simulink model "MEKFTester"  (R2025b)
settings: Solver=VariableStepAuto  StartTime=0.0  StopTime=2000  RelTol=1e-3
values from neighbouring files (symbols this model uses):
  F = StateTransitionMat(z(1:3), z(4:6), R_b2i)    [EstimateStateFCN.m]    (also in FlightEstimator.m = StateTransitionMat(z(1:3), z(4:6), R_b2i, 0); GroundEstimator.m = StateTransitionMat(z(1:3), z(4:6), R_b2i, 1); StateTransitionMat.m = zeros(15))
  q = q / norm(q)    [EstimateStateFCN.m]    (also in FlightEstimator.m; GroundEstimator.m)
undefined symbols (not defined in the file or in its folder): constantsASTRA, DiscIntNeverNeededParam, distMode, dt_SIM, IMU_Rate, Light, magDistMatrix, MIL, u0, x0
libraries: aerolibnav x2, aerolibwind2 x1, simulink x1
settings Model: PacingRate=5  Creator=antho  LastModifiedBy=pplat

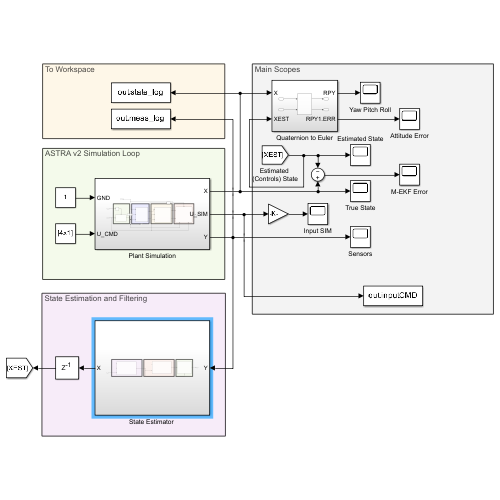
[thumbnail: Simulink's stored preview of the top-level diagram]
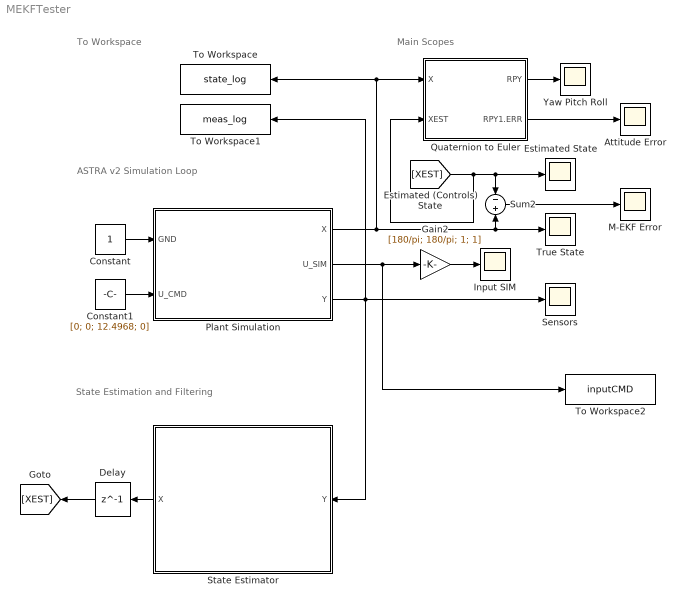
== system MEKFTester ==
  note: To Workspace
  note: Main Scopes
  note: State Estimation and Filtering
  note: ASTRA v2 Simulation Loop
  Attitude Error : Scope
      settings: ActiveDisplayYMinimum=-3.1070378293328353  ActiveDisplayYMaximum=3.3991083276723568  DataLoggingVariableName=ScopeData9
  Constant : Constant
  Constant1 : Constant  Value=[0; 0; 12.4968; 0]
  Delay : Delay  DelayLength=1  InitialCondition=[1; zeros(18,1)]
  Estimated State : Scope
      settings: ActiveDisplayYMinimum=0.77321879382653858  ActiveDisplayYMaximum=0.79869453057358752
  Gain2 : Gain  Gain=[180/pi; 180/pi; 1; 1]
  Input SIM : Scope
      settings: ActiveDisplayYMinimum=-0.41301379982025921  ActiveDisplayYMaximum=0.5556666783325932  DataLoggingVariableName=ScopeData4
  M-EKF Error : Scope
      settings: ActiveDisplayYMinimum=-0.21315959179084651  ActiveDisplayYMaximum=0.079913819904229133  DataLoggingVariableName=ScopeData2
  Plant Simulation : Subsystem
  Quaternion to Euler : Subsystem
  Sensors : Scope
      settings: ActiveDisplayYMinimum=-2.5727575775910978  ActiveDisplayYMaximum=2.4937672733000804  DataLoggingVariableName=ScopeData3
  "State Estimator " : Subsystem
  Sum2 : Sum  Inputs=-|+
  To Workspace : ToWorkspace  VariableName=state_log  SaveFormat=Timeseries  SampleTime=-1
  To Workspace1 : ToWorkspace  VariableName=meas_log  SaveFormat=Timeseries  SampleTime=-1
  To Workspace2 : ToWorkspace  VariableName=inputCMD  SaveFormat=Timeseries  SampleTime=-1
  True State : Scope
      settings: ActiveDisplayYMinimum=-1.2379536808786333  ActiveDisplayYMaximum=1.2486615200976259
  Yaw Pitch Roll : Scope
      settings: ActiveDisplayYMinimum=-224.99023889502547  ActiveDisplayYMaximum=224.99733749831469  DataLoggingVariableName=ScopeData7
  wires:
  [XEST] -> Quaternion to Euler/2(XEST), Sum2/1, Estimated State/1
  Sum2/1 -> M-EKF Error/1
  Delay/1 -> [XEST]
  Gain2/1 -> Input SIM/1
  Plant Simulation/2(U_SIM) -> To Workspace2/1, Gain2/1
  Quaternion to Euler/1(RPY) -> Yaw Pitch Roll/1
  Plant Simulation/3(Y) -> Sensors/1, "State Estimator "/1(Y), To Workspace1/1
  Plant Simulation/1(X) -> Sum2/2, True State/1, Quaternion to Euler/1(X), To Workspace/1
  Constant/1 -> Plant Simulation/1(GND)
  Constant1/1 -> Plant Simulation/2(U_CMD)
  "State Estimator "/1(X) -> Delay/1
  Quaternion to Euler/2(RPY1.ERR) -> Attitude Error/1

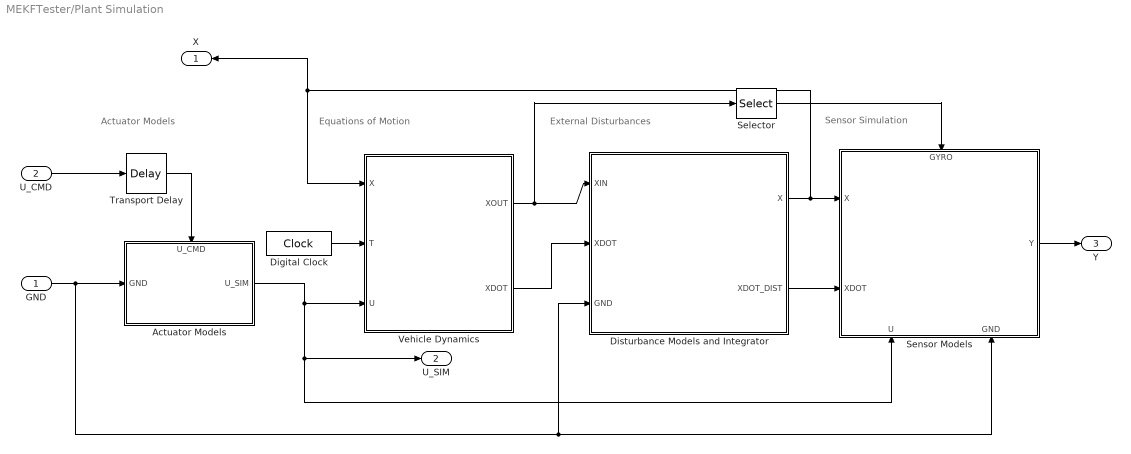
== system MEKFTester/Plant Simulation ==
  note: Equations of Motion
  note: Actuator Models
  note: External Disturbances
  note: Sensor Simulation
  GND : Inport
  U_CMD : Inport  Port=2
  Actuator Models : Subsystem
      settings: PortSchema="{\"entries\":[{\"content\":{\"sides\":[{\"content\":{\"connectorIds\":[\"In1\"]},\"type\":\"ConnectorPlacement.EquallySpacedRectSide\",\"uuid\":\"54343072-6023-41e9-a0f6-81f6bed17e05\"},{\"content\":{\"connectorIds\":[\"Out1\"],\"side\":\"RIGHT\"},\"type\":\"ConnectorPlacement.EquallySpacedRectSide\",\"uuid\":\"2ed3290f-d38b-41d8-95ae-d88068502334\"},{\"content\":{\"connectorIds\":[\"In2\"],\"side\":\"TOP\"},\"type\":\"ConnectorPlacement.EquallySpacedRectSide\",\"uuid\":\"e9e41c57-b871-4be2-92e8-dfbbf995d6b0\"}]},\"type\":\"ConnectorPlacement.EquallySpacedConnector\",\"uuid\":\"c037521e-b20b-40c6-bb74-3aafe8fc1476\"}],\"packageUris\":[\"http://schema.mathworks.com/mf0/Connector/R2020b\"],\"version\":\"1.0\"}"
  Digital Clock : DigitalClock  SampleTime=dt_SIM
  Disturbance Models and Integrator : Subsystem
  Selector : Selector  InputPortWidth=19  IndexOptions=Index vector (dialog)  Indices=[11:13]  OutputSizes=1
  Sensor Models : Subsystem
      settings: PortSchema="{\"entries\":[{\"content\":{\"sides\":[{\"content\":{\"connectorIds\":[\"In1\",\"In2\"]},\"type\":\"ConnectorPlacement.EquallySpacedRectSide\",\"uuid\":\"9bc4a206-bba4-4c50-88a9-89b0392ab722\"},{\"content\":{\"connectorIds\":[\"Out1\"],\"side\":\"RIGHT\"},\"type\":\"ConnectorPlacement.EquallySpacedRectSide\",\"uuid\":\"162bbd17-e1b8-4f29-9191-53e17e38d79d\"},{\"content\":{\"connectorIds\":[\"In3\"],\"side\":\"TOP\"},\"type\":\"ConnectorPlacement.EquallySpacedRectSide\",\"uuid\":\"c56a23db-6a5c-435f-99fd-d50fc9dbdc94\"},{\"content\":{\"connectorIds\":[\"In4\",\"In5\"],\"side\":\"BOTTOM\"},\"type\":\"ConnectorPlacement.EquallySpacedRectSide\",\"uuid\":\"e0c2a0dc-3b7a-40ac-8345-28e7bf7b9405\"}]},\"type\":\"ConnectorPlacement.EquallySpacedConnector\",\"uuid\":\"d1c29f55-9be5-4f45-9d70-06beba2c2f44\"}],\"packageUris\":[\"http://schema.mathworks.com/mf0/Connector/R2020b\"],\"version\":\"1.0\"}"
  Transport Delay : TransportDelay  DelayTime=0.02  InitialOutput=u0
  Vehicle Dynamics : Subsystem
  X : Outport
  U_SIM : Outport  Port=2
  Y : Outport  Port=3
  wires:
  Vehicle Dynamics/2(XDOT) -> Disturbance Models and Integrator/2(XDOT)
  Sensor Models/1(Y) -> Y/1
  GND/1 -> Actuator Models/1(GND), Sensor Models/5(GND), Disturbance Models and Integrator/3(GND)
  Disturbance Models and Integrator/1(X) -> Vehicle Dynamics/1(X), X/1, Sensor Models/1(X)
  Disturbance Models and Integrator/2(XDOT_DIST) -> Sensor Models/2(XDOT)
  Actuator Models/1(U_SIM) -> U_SIM/1, Sensor Models/4(U), Vehicle Dynamics/3(U)
  U_CMD/1 -> Transport Delay/1
  Transport Delay/1 -> Actuator Models/2(U_CMD)
  Vehicle Dynamics/1(XOUT) -> Selector/1, Disturbance Models and Integrator/1(XIN)
  Digital Clock/1 -> Vehicle Dynamics/2(T)
  Selector/1 -> Sensor Models/3(GYRO)

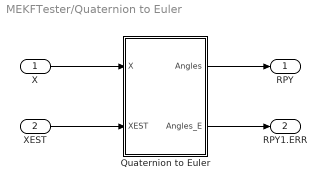
== system MEKFTester/Quaternion to Euler ==
  X : Inport
  XEST : Inport  Port=2
  Quaternion to Euler : MATLAB Function  TreatAsAtomicUnit=on
  RPY : Outport
  RPY1.ERR : Outport  Port=2
  wires:
  X/1 -> Quaternion to Euler/1(X)
  Quaternion to Euler/1(Angles) -> RPY/1
  XEST/1 -> Quaternion to Euler/2(XEST)
  Quaternion to Euler/2(Angles_E) -> RPY1.ERR/1

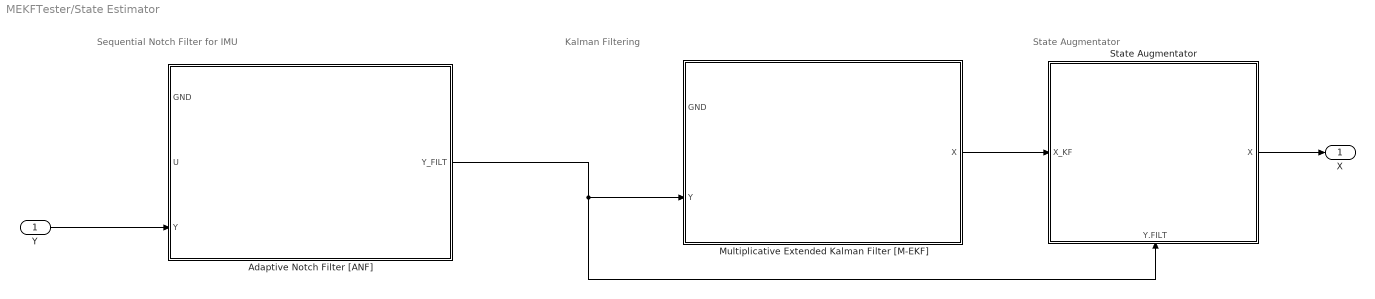
== system MEKFTester/State Estimator  ==
  note: Sequential Notch Filter for IMU
  note: State Augmentator
  note: Kalman Filtering
  Y : Inport
  Adaptive Notch Filter [ANF] : Subsystem
  Multiplicative Extended Kalman Filter [M-EKF] : Subsystem
  State Augmentator : Subsystem
      settings: PortSchema="{\"entries\":[{\"content\":{\"sides\":[{\"content\":{\"connectorIds\":[\"In1\"]},\"type\":\"ConnectorPlacement.EquallySpacedRectSide\",\"uuid\":\"bb6458aa-622a-4d42-b468-f616d6e302fe\"},{\"content\":{\"connectorIds\":[\"Out1\"],\"side\":\"RIGHT\"},\"type\":\"ConnectorPlacement.EquallySpacedRectSide\",\"uuid\":\"af8bade2-eb0a-4714-9db5-d33244eb3558\"},{\"content\":{\"side\":\"TOP\"},\"type\":\"ConnectorPlacement.EquallySpacedRectSide\",\"uuid\":\"05a7f106-e447-475e-b3b5-727cb0579a7b\"},{\"content\":{\"connectorIds\":[\"In2\"],\"side\":\"BOTTOM\"},\"type\":\"ConnectorPlacement.EquallySpacedRectSide\",\"uuid\":\"a6d44455-a42d-44f7-b37b-0d3db398c8f2\"}]},\"type\":\"ConnectorPlacement.EquallySpacedConnector\",\"uuid\":\"c6f62579-6b17-43b5-92f1-6190f0d9fd8b\"}],\"packageUris\":[\"http://schema.mathworks.com/mf0/Connector/R2020b\"],\"version\":\"1.0\"}"
  X : Outport
  wires:
  Multiplicative Extended Kalman Filter [M-EKF]/1(X) -> State Augmentator/1(X_KF)
  State Augmentator/1(X) -> X/1
  Adaptive Notch Filter [ANF]/1(Y_FILT) -> State Augmentator/2(Y.FILT), Multiplicative Extended Kalman Filter [M-EKF]/2(Y)
  Y/1 -> Adaptive Notch Filter [ANF]/3(Y)

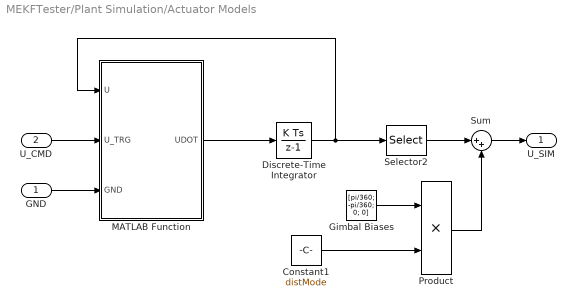
== system MEKFTester/Plant Simulation/Actuator Models ==
  GND : Inport
  U_CMD : Inport  Port=2
  Constant1 : Constant  Value=distMode
  Discrete-Time Integrator : DiscreteIntegrator  InitialCondition=[zeros(4,1); u0(3); 0]  SampleTime=-1  ICPrevOutput=DiscIntNeverNeededParam  ICPrevScaledInput=DiscIntNeverNeededParam
  Gimbal Biases : Constant  Value=[pi/360; -pi/360; 0; 0]
  MATLAB Function : MATLAB Function  TreatAsAtomicUnit=on
  Product : Product
  Selector2 : Selector  InputPortWidth=6  IndexOptions=Index vector (dialog)  Indices=[1 3 5 6]  OutputSizes=1
  Sum : Sum  Inputs=|++
  U_SIM : Outport
  wires:
  U_CMD/1 -> MATLAB Function/2(U_TRG)
  MATLAB Function/1(UDOT) -> Discrete-Time Integrator/1
  Discrete-Time Integrator/1 -> MATLAB Function/1(U), Selector2/1
  GND/1 -> MATLAB Function/3(GND)
  Sum/1 -> U_SIM/1
  Selector2/1 -> Sum/1
  Gimbal Biases/1 -> Product/1
  Product/1 -> Sum/2
  Constant1/1 -> Product/2

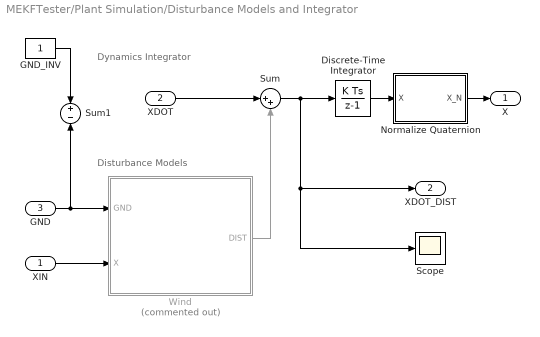
== system MEKFTester/Plant Simulation/Disturbance Models and Integrator ==
  note: Disturbance Models
  note: Dynamics Integrator
  XIN : Inport
  XDOT : Inport  Port=2
  GND : Inport  Port=3
  Discrete-Time Integrator : DiscreteIntegrator  InitialCondition=[x0; zeros(3,1)]  SampleTime=-1  ICPrevOutput=DiscIntNeverNeededParam  ICPrevScaledInput=DiscIntNeverNeededParam
  GND_INV : Constant
  Normalize Quaternion : MATLAB Function  TreatAsAtomicUnit=on
  Scope : Scope
      settings: ActiveDisplayYMinimum=-1  ActiveDisplayYMaximum=1  DataLoggingVariableName=ScopeData8
  Sum : Sum  Inputs=|++
  Sum1 : Sum  Inputs=+|-
  Wind : Subsystem  Commented=on
  X : Outport
  XDOT_DIST : Outport  Port=2
  wires:
  Discrete-Time Integrator/1 -> Normalize Quaternion/1(X)
  XIN/1 -> Wind/2(X)
  Wind/1(DIST) -> Sum/2
  GND_INV/1 -> Sum1/1
  GND/1 -> Wind/1(GND), Sum1/2
  XDOT/1 -> Sum/1
  Sum/1 -> Discrete-Time Integrator/1, Scope/1, XDOT_DIST/1
  Normalize Quaternion/1(X_N) -> X/1

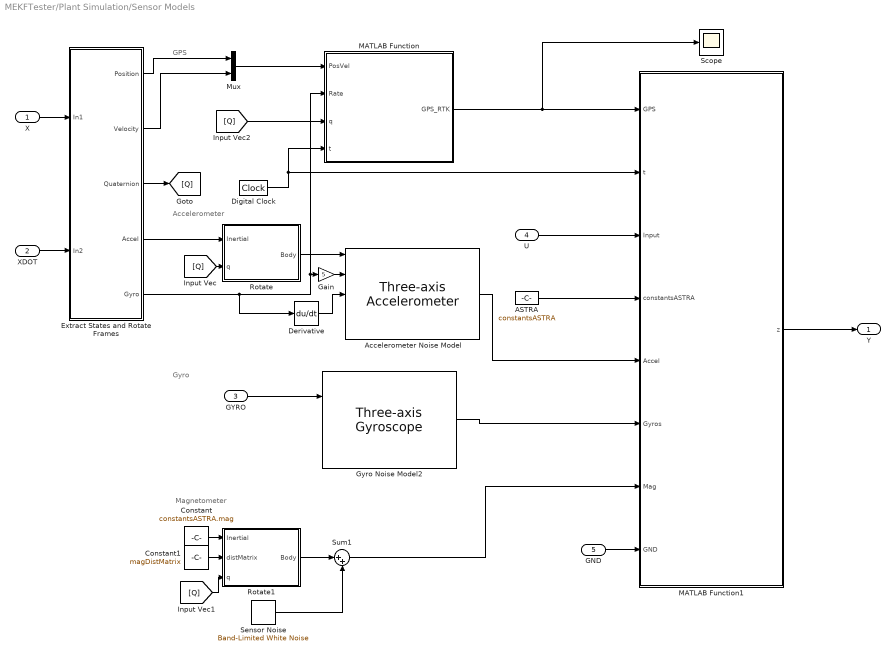
== system MEKFTester/Plant Simulation/Sensor Models ==
  note: Gyro
  note: Accelerometer
  note: Magnetometer
  note: GPS
  X : Inport
  XDOT : Inport  Port=2
  GYRO : Inport  Port=3
  U : Inport  Port=4
  GND : Inport  Port=5
  ASTRA : Constant  Value=constantsASTRA  OutDataTypeStr=Bus: slBus1
  Accelerometer Noise Model : aerolibnav/Three-axis Accelerometer  units=Metric (MKS)  acc=[0 0 0.3]  gtype=on  dtype_a=on  w_a=190  z_a=0.707  a_sf_cc=eye(3)  a_bias=accelBias  a_Ts=1 / IMU_Rate  a_rand=on  a_seeds=[23093 23094 23095]  a_pow=ones(1,3) * 0.09^2 * 1 / IMU_Rate  a_sat="[-inf  -inf  -inf  inf inf inf]"
  Constant : Constant  Value=constantsASTRA.mag
  Constant1 : Constant  Value=magDistMatrix
  Derivative : Derivative
  Digital Clock : DigitalClock  SampleTime=dt_SIM
  Extract States and Rotate Frames : Subsystem
  Gain : Gain  Gain=5
  Gyro Noise Model2 : aerolibnav/Three-axis Gyroscope  dtype_g=on  w_g=190  z_g=0.707  g_sf_cc=eye(3)  g_bias=gyroBias  g_sen=0  g_Ts=1 / IMU_Rate  g_rand=on  g_seeds=[23093 23094 23095]  g_pow=ones(1,3) * 0.05^2 * 1 / IMU_Rate  g_sat="[-inf  -inf  -inf  inf inf inf]"
  MATLAB Function : MATLAB Function  TreatAsAtomicUnit=on
  MATLAB Function1 : MATLAB Function  TreatAsAtomicUnit=on
  Mux : Mux  Inputs=2
  Rotate : MATLAB Function  TreatAsAtomicUnit=on
  Rotate1 : MATLAB Function  TreatAsAtomicUnit=on
  Scope : Scope
      settings: ActiveDisplayYMinimum=-1  ActiveDisplayYMaximum=1  DataLoggingVariableName=ScopeData10
  Sensor Noise : simulink/Sources/Band-Limited White Noise  Cov=(2E-2)^2  Ts=dt_SIM  seed=[23341,23342,23343]
  Sum1 : Sum  Inputs=|++
  Y : Outport
  wires:
  X/1 -> Extract States and Rotate Frames/1(In1)
  XDOT/1 -> Extract States and Rotate Frames/2(In2)
  Digital Clock/1 -> MATLAB Function/4(t), MATLAB Function1/2(t)
  Extract States and Rotate Frames/5(Gyro) -> Derivative/1, Gain/1, MATLAB Function/2(Rate)
  Extract States and Rotate Frames/3(Quaternion) -> [Q]
  Rotate/1(Body) -> Accelerometer Noise Model/1
  Extract States and Rotate Frames/4(Accel) -> Rotate/1(Inertial)
  [Q] -> Rotate/2(q)
  Constant/1 -> Rotate1/1(Inertial)
  [Q] -> Rotate1/3(q)
  Sensor Noise/1 -> Sum1/2
  Rotate1/1(Body) -> Sum1/1
  Sum1/1 -> MATLAB Function1/7(Mag)
  MATLAB Function/1(GPS_RTK) -> Scope/1, MATLAB Function1/1(GPS)
  Accelerometer Noise Model/1 -> MATLAB Function1/5(Accel)
  Gyro Noise Model2/1 -> MATLAB Function1/6(Gyros)
  MATLAB Function1/1(z) -> Y/1
  ASTRA/1 -> MATLAB Function1/4(constantsASTRA)
  Extract States and Rotate Frames/2(Velocity) -> Mux/2
  Mux/1 -> MATLAB Function/1(PosVel)
  Extract States and Rotate Frames/1(Position) -> Mux/1
  U/1 -> MATLAB Function1/3(Input)
  GND/1 -> MATLAB Function1/8(GND)
  Constant1/1 -> Rotate1/2(distMatrix)
  [Q] -> MATLAB Function/3(q)
  GYRO/1 -> Gyro Noise Model2/1
  Gain/1 -> Accelerometer Noise Model/2
  Derivative/1 -> Accelerometer Noise Model/3

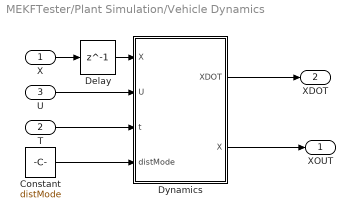
== system MEKFTester/Plant Simulation/Vehicle Dynamics ==
  X : Inport
  T : Inport  Port=2
  U : Inport  Port=3
  Constant : Constant  Value=distMode
  Delay : Delay  DelayLength=1  InitialCondition=[x0; zeros(3,1)]
  Dynamics : MATLAB Function  TreatAsAtomicUnit=on
  XOUT : Outport
  XDOT : Outport  Port=2
  wires:
  Dynamics/1(XDOT) -> XDOT/1
  U/1 -> Dynamics/2(U)
  X/1 -> Delay/1
  Constant/1 -> Dynamics/4(distMode)
  Dynamics/2(X) -> XOUT/1
  T/1 -> Dynamics/3(t)
  Delay/1 -> Dynamics/1("X ")

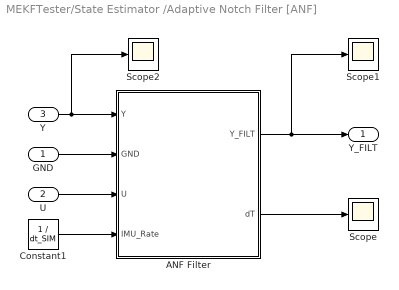
== system MEKFTester/State Estimator /Adaptive Notch Filter [ANF] ==
  GND : Inport
  U : Inport  Port=2
  Y : Inport  Port=3
  ANF Filter : MATLAB Function  TreatAsAtomicUnit=on
  Constant1 : Constant  Value=1 / dt_SIM
  Scope : Scope
      settings: ActiveDisplayYMinimum=0.00097880622837365075  ActiveDisplayYMaximum=0.0020384948096911198  DataLoggingVariableName=ScopeData12
  Scope1 : Scope
      settings: ActiveDisplayYMinimum=9.4335953871319269  ActiveDisplayYMaximum=11.786797462805113  DataLoggingVariableName=ScopeData15
  Scope2 : Scope
      settings: ActiveDisplayYMinimum=-0.822722965610661  ActiveDisplayYMaximum=0.985135629551039  DataLoggingVariableName=ScopeData16
  Y_FILT : Outport
  wires:
  ANF Filter/1(Y_FILT) -> Scope1/1, Y_FILT/1
  GND/1 -> ANF Filter/2(GND)
  U/1 -> ANF Filter/3(U)
  Y/1 -> Scope2/1, ANF Filter/1(Y)
  Constant1/1 -> ANF Filter/4(IMU_Rate)
  ANF Filter/2(dT) -> Scope/1

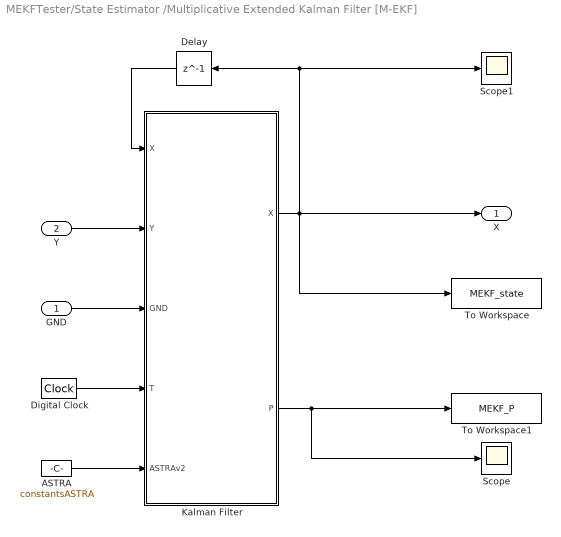
== system MEKFTester/State Estimator /Multiplicative Extended Kalman Filter [M-EKF] ==
  GND : Inport
  Y : Inport  Port=2
  ASTRA : Constant  Value=constantsASTRA  OutDataTypeStr=Bus: slBus1
  Delay : Delay  DelayLength=1  InitialCondition=[1; zeros(18,1)]
  Digital Clock : DigitalClock  SampleTime=dt_SIM
  Kalman Filter : MATLAB Function  TreatAsAtomicUnit=on
  Scope : Scope
      settings: ActiveDisplayYMinimum=-0.020501461331404704  ActiveDisplayYMaximum=0.18451803346425907  DataLoggingVariableName=ScopeData17
  Scope1 : Scope
      settings: ActiveDisplayYMinimum=-0.52078107403838736  ActiveDisplayYMaximum=0.65910315182601131  DataLoggingVariableName=ScopeData11
  To Workspace : ToWorkspace  VariableName=MEKF_state  SaveFormat=Timeseries  SampleTime=-1
  To Workspace1 : ToWorkspace  VariableName=MEKF_P  SaveFormat=Timeseries  SampleTime=-1
  X : Outport
  wires:
  Digital Clock/1 -> Kalman Filter/4(T)
  Kalman Filter/1(X) -> To Workspace/1, Scope1/1, Delay/1, X/1
  Y/1 -> Kalman Filter/2(Y)
  Delay/1 -> Kalman Filter/1("X ")
  ASTRA/1 -> Kalman Filter/5(ASTRAv2)
  GND/1 -> Kalman Filter/3(GND)
  Kalman Filter/2(P) -> Scope/1, To Workspace1/1

== system MEKFTester/State Estimator /State Augmentator ==
  X_KF : Inport
  Y.FILT : Inport  Port=2
  MATLAB Function : MATLAB Function  TreatAsAtomicUnit=on
  X : Outport
  wires:
  X_KF/1 -> MATLAB Function/1(XKF)
  MATLAB Function/1(X) -> X/1
  Y.FILT/1 -> MATLAB Function/2(Y)

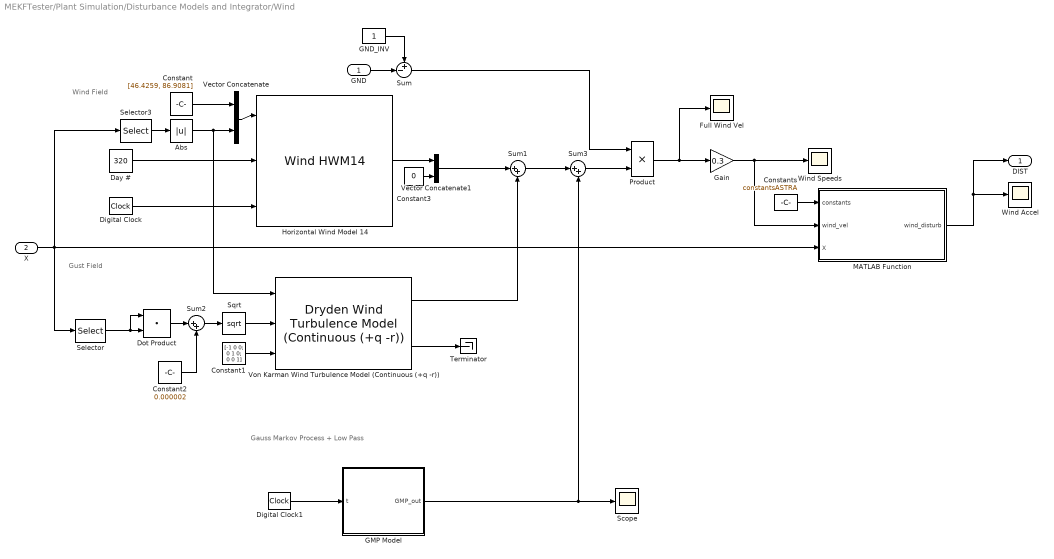
== system MEKFTester/Plant Simulation/Disturbance Models and Integrator/Wind ==
  note: Gauss Markov Process + Low Pass
  note: Gust Field
  note: Wind Field
  GND : Inport
  X : Inport  Port=2
  Abs : Abs  SaturateOnIntegerOverflow=off
  Constant : Constant  Value=[46.4259, 86.9081]
  Constant1 : Constant  Value=[-1 0 0; 0 1 0; 0 0 1]
  Constant2 : Constant  Value=0.000002
  Constant3 : Constant  Value=0
  Constants : Constant  Value=constantsASTRA  OutDataTypeStr=Bus: slBus1
  Day # : Constant  Value=320
  Digital Clock : DigitalClock  SampleTime=dt_SIM
  Digital Clock1 : DigitalClock  SampleTime=dt_SIM
  Dot Product : DotProduct  OutDataTypeStr=Inherit: Inherit via internal rule
  Full Wind Vel : Scope
      settings: ActiveDisplayYMinimum=-5.9330847029288414  ActiveDisplayYMaximum=4.4700897462030218  DataLoggingVariableName=ScopeData13
  GMP Model : MATLAB Function  TreatAsAtomicUnit=on
  GND_INV : Constant
  Gain : Gain  Gain=0.3
  Horizontal Wind Model 14 : WindHWM14
  MATLAB Function : MATLAB Function  TreatAsAtomicUnit=on
  Product : Product
  Scope : Scope
      settings: ActiveDisplayYMinimum=-2.8676060433464485  ActiveDisplayYMaximum=2.8612107779538238  DataLoggingVariableName=ScopeData14
  Selector : Selector  InputPortWidth=16  IndexOptions=Index vector (dialog)  Indices=[8:10]  OutputSizes=1
  Selector3 : Selector  InputPortWidth=16  IndexOptions=Index vector (dialog)  Indices=7  OutputSizes=1
  Sqrt : Sqrt
  Sum : Sum  Inputs=+-|
  Sum1 : Sum  Inputs=|++
  Sum2 : Sum  Inputs=|++
  Sum3 : Sum  Inputs=|++
  Terminator : Terminator
  Vector Concatenate : Concatenate
  Vector Concatenate1 : Concatenate
  Von Karman Wind Turbulence Model (Continuous (+q -r)) : aerolibwind2/Dryden Wind Turbulence Model  (Continuous (+q -r))  units=Metric (MKS)  spec=MIL-F-8785C  model=Continuous Von Karman (+q -r)  W20=15  Wdeg=0  TurbProb=10^-2 - Light  L_high=762  Wingspan=10  ts=0.1  Seed=[23341 23342 23343 23344]  T_on=on
      settings: LibrarySourceBlock=|
      | aerolibwind2/Von Karman Wind Turbulence Model
      | (Continuous (+q -r))
  Wind Accel : Scope
      settings: ActiveDisplayYMinimum=-0.93847040858698449  ActiveDisplayYMaximum=0.85102417935944119  DataLoggingVariableName=ScopeData5
  Wind Speeds : Scope
      settings: ActiveDisplayYMinimum=-6.0032131159962416  ActiveDisplayYMaximum=4.44789373969359  DataLoggingVariableName=ScopeData5
  DIST : Outport
  wires:
  Digital Clock/1 -> Horizontal Wind Model 14/3
  Day #/1 -> Horizontal Wind Model 14/2
  MATLAB Function/1(wind_disturb) -> DIST/1, Wind Accel/1
  Vector Concatenate/1 -> Horizontal Wind Model 14/1
  Selector3/1 -> Abs/1
  Constant/1 -> Vector Concatenate/1
  GND/1 -> Sum/2
  Sum/1 -> Product/1
  GND_INV/1 -> Sum/1
  Horizontal Wind Model 14/1 -> Vector Concatenate1/1
  Constants/1 -> MATLAB Function/1(constants)
  Selector/1 -> Dot Product/1, Dot Product/2
  Sqrt/1 -> Von Karman Wind Turbulence Model (Continuous (+q -r))/2
  Von Karman Wind Turbulence Model (Continuous (+q -r))/1 -> Sum1/2
  Constant1/1 -> Von Karman Wind Turbulence Model (Continuous (+q -r))/3
  Sum2/1 -> Sqrt/1
  Dot Product/1 -> Sum2/1
  Constant2/1 -> Sum2/2
  X/1 -> Selector3/1, MATLAB Function/3(X), Selector/1
  Abs/1 -> Vector Concatenate/2, Von Karman Wind Turbulence Model (Continuous (+q -r))/1
  Product/1 -> Full Wind Vel/1, Gain/1
  Vector Concatenate1/1 -> Sum1/1
  Constant3/1 -> Vector Concatenate1/2
  Von Karman Wind Turbulence Model (Continuous (+q -r))/2 -> Terminator/1
  Gain/1 -> Wind Speeds/1, MATLAB Function/2(wind_vel)
  Sum3/1 -> Product/2
  Sum1/1 -> Sum3/1
  GMP Model/1(GMP_out) -> Scope/1, Sum3/2
  Digital Clock1/1 -> GMP Model/1(t)

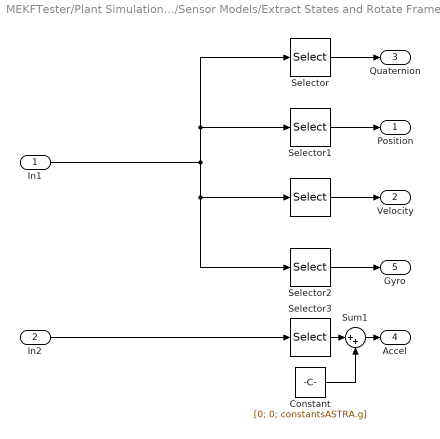
== system MEKFTester/Plant Simulation/Sensor Models/Extract States and Rotate Frames ==
  In1 : Inport
  In2 : Inport  Port=2
  "  " : Selector  InputPortWidth=19  IndexOptions=Index vector (dialog)  Indices=[8:10]  OutputSizes=1
  Constant : Constant  Value=[0; 0; constantsASTRA.g]
  Selector : Selector  InputPortWidth=19  IndexOptions=Index vector (dialog)  Indices=[1:4]  OutputSizes=1
  Selector1 : Selector  InputPortWidth=19  IndexOptions=Index vector (dialog)  Indices=[5:7]  OutputSizes=1
  Selector2 : Selector  InputPortWidth=19  IndexOptions=Index vector (dialog)  Indices=[11:13]  OutputSizes=1
  Selector3 : Selector  InputPortWidth=19  IndexOptions=Index vector (dialog)  Indices=[8:10]  OutputSizes=1
  Sum1 : Sum  Inputs=|++
  Position : Outport
  Velocity : Outport  Port=2
  Quaternion : Outport  Port=3
  Accel : Outport  Port=4
  Gyro : Outport  Port=5
  wires:
  Selector/1 -> Quaternion/1
  Selector1/1 -> Position/1
  "  "/1 -> Velocity/1
  Selector2/1 -> Gyro/1
  Selector3/1 -> Sum1/1
  Sum1/1 -> Accel/1
  Constant/1 -> Sum1/2
  In1/1 -> Selector1/1, Selector/1, Selector2/1, "  "/1
  In2/1 -> Selector3/1

== matlab function MEKFTester/Plant Simulation/Sensor Models/MATLAB Function1 ==
  data: GPS input; t input; Input input; constantsASTRA input; Accel input; z output; Gyros input; Mag input; GND input
function z = SensorFrequency(GPS, t, Input, constantsASTRA, Accel, Gyros, Mag, GND)
%% Add Thrust Varying Oscillation
persistent phase lastT
if isempty(phase)
    phase = 0;
    lastT = 0;
end
dt = t - lastT;
lastT = t;

% Thrust vibration generator
Track = [1.3525    42.6278];
THRUST = Input(3) / constantsASTRA.MaxT * 100;
w = 2 * pi * (Track(1) * THRUST + Track(2) + 1 * randn());
phase = phase + w * dt;
MaxAmplAccel = 7;
MaxAmplGyro = 0.2;
Accel = Accel + MaxAmplAccel * THRUST / 100 * sin(phase) * (1 - GND);
Gyros = Gyros + MaxAmplGyro * THRUST / 100 * sin(phase) * (1 - GND);
z = [Accel; Gyros; Mag; GPS];

== matlab function MEKFTester/Plant Simulation/Disturbance Models and Integrator/Wind/GMP Model ==
  data: t input; GMP_out output
function GMP_out = GMP(t)

persistent errorval lastTime EMA
if isempty(errorval)
    errorval = 0;
    EMA = 0;
    lastTime = 0;  % Update last timestamp
end

dT = t - lastTime;

% First order Gauss Markov Process for additional disturbance
decay = 10;
beta = exp(-dT / decay);
covar = 1;
errorval = beta * errorval + sqrt(1 - beta^2) * covar * randn;

% EMA Step to kill High Freq. Noise
EMA = ExpMovingAvg(errorval, EMA, 0.05);
GMP_out = EMA * ones(3,1);
lastTime = t;

== matlab function MEKFTester/State Estimator /Adaptive Notch Filter [ANF]/ANF Filter ==
  data: Y input; Y_FILT output; GND input; U input; IMU_Rate input; dT output
function [Y_FILT, dT] = ANF_Filter(Y, GND, U, IMU_Rate)

% Extract IMU
IMU = Y(1:9);
dT = 1 / IMU_Rate;

% Thrust PCT
% THRUST = U(3) / (1.697 * 9.80145) * 100;

% ANF Filter
ANF_IMU = DigitalNF(IMU, 1, 0, dT);

% Combine (FILTER CURRENTLY OFF)
Y_FILT = [ANF_IMU; Y(10:15)];

== matlab function MEKFTester/Plant Simulation/Vehicle Dynamics/Dynamics ==
  data: X input; XDOT output; U input; t input; distMode input; X output
function [XDOT, X] = Dynamics(X, U, t, distMode)

persistent errorval lastTime EMA
if isempty(errorval)
    errorval = zeros(3,1);
    EMA = zeros(3,1);
    lastTime = 0;  % Update last timestamp
end

dT = t - lastTime;

% First order Gauss Markov Process for additional disturbance
decay = 5;
beta = exp(-dT / decay);
covar = 0.6;
errorval = beta * errorval + sqrt(1 - beta^2) * covar * randn(3,1);

% EMA Step to kill High Freq. Noise
EMA = ExpMovingAvg(errorval, EMA, 0.05);
GMP_out = EMA;
lastTime = t;
X(11:13) = GMP_out;
q = X(1:4);
M = [q(1) -q(2) -q(3) -q(4);
     q(2)  q(1) -q(4)  q(3);
     q(3)  q(4)  q(1) -q(2);
     q(4) -q(3)  q(2)  q(1)];
QDOT = 0.5 * M * [0; X(11:13)];
XDOT = [QDOT; zeros(15,1)];

% if distMode == 1
%     XDOT = disturbedDynamics(X, U);
% else
%     XDOT = nominalDynamics(X, U);
% end

== matlab function MEKFTester/Plant Simulation/Sensor Models/Rotate ==
  data: Inertial input; Body output; q input
function Body = Rotate(Inertial, q)
Body = quatRot(q) * Inertial;

== matlab function MEKFTester/State Estimator /Multiplicative Extended Kalman Filter [M-EKF]/Kalman Filter ==
  data: X input; Y input; GND input; X output; T input; ASTRAv2 input; P output
function [X, P] = MEKF(X, Y, GND, T, ASTRAv2)

    % Measure simulation timestep
    persistent dt lastT lastP
    if isempty(dt)
        dt = 0;
        lastT = 0;
        lastP = eye(18);
    end
    dt = T - lastT;
    lastT = T;
    
    if true
        [X, lastP] = GroundEstimator(X, ASTRAv2, Y, dt);
    else
        [X, lastP(1:9, 1:9)] = FlightEstimator(X, ASTRAv2, Y, dt, lastP(1:9, 1:9));
    end
    P = diag(lastP);
end
    %X = EstimateStateFCN(X, ASTRAv2, Y, dt, GND);

== matlab function MEKFTester/Plant Simulation/Disturbance Models and Integrator/Wind/MATLAB Function ==
  data: constants input; wind_vel input; X input; wind_disturb output
function wind_disturb = wind_sim(constants, wind_vel, X)

wind_disturb = wind(constants, wind_vel, X);

== matlab function MEKFTester/Plant Simulation/Actuator Models/MATLAB Function ==
  data: U input; UDOT output; U_TRG input; GND input
function UDOT = Actuators(U, U_TRG, GND)

    UDOT = ActuatorDynamics(U, U_TRG, GND);
end

== matlab function MEKFTester/Quaternion to Euler/Quaternion to Euler ==
  data: X input; Angles output; XEST input; Angles_E output
function [Angles, Angles_E] = q2eul(X, XEST)

% Complete quaternion & error quaternion
q = X(1:4);
qest = XEST(1:4);

Q_Conj = [qest(1); -qest(2:4)];
qerr = HamiltonianProd(Q_Conj) * q;
if qerr(1) < 0
    qerr = -qerr;
end

% Quaternion to Euler Angles
Roll = atan2(2*(q(1) * q(2) + q(3) * q(4)), 1 - 2*(q(2)^2 + q(3)^2));
Pitch = asin(2*(q(1) * q(3) - q(4) * q(2)));
Yaw = atan2(2*(q(1) * q(4) + q(2) * q(3)), 1 - 2*(q(3)^2 + q(4)^2));

% Error Euler Angles
Roll_E = atan2(2*(qerr(1) * qerr(2) + qerr(3) * qerr(4)), 1 - 2*(qerr(2)^2 + qerr(3)^2));
Pitch_E = asin(2*(qerr(1) * qerr(3) - qerr(4) * qerr(2)));
Yaw_E = atan2(2*(qerr(1) * qerr(4) + qerr(2) * qerr(3)), 1 - 2*(qerr(3)^2 + qerr(4)^2));


% Angle Vector
Angles = [Roll; Pitch; Yaw] * 180/pi;
Angles_E = [Roll_E; Pitch_E; Yaw_E] * 180/pi;

== matlab function MEKFTester/State Estimator /State Augmentator/MATLAB Function ==
  data: XKF input; X output; Y input
function X = StateAUG(XKF, Y)

% Change Filter State to Controls State
X = [XKF(1:4); XKF(5:7); XKF(8:10); Y(4:6) - XKF(11:13); XKF(11:13); XKF(14:16)];

== matlab function MEKFTester/Plant Simulation/Disturbance Models and Integrator/Normalize Quaternion ==
  data: X input; X_N output
function X_N = fcn(X)
X_N = [X(1:4) / norm(X(1:4)); X(5:end)];

== matlab function MEKFTester/Plant Simulation/Sensor Models/Rotate1 ==
  data: Inertial input; distMatrix input; Body output; q input
function Body = Rotate(Inertial, distMatrix, q)
S = 53.5;
distMatrix = eye(3);
Body = quatRot(q) * distMatrix * (S * Inertial) + 5 * ones(3,1);

== matlab function MEKFTester/Plant Simulation/Sensor Models/MATLAB Function ==
  data: PosVel input; Rate input; q input; GPS_RTK output; t input
function GPS_RTK = GPS(PosVel, Rate, q, t)

R_b2i = quatRot(q)';
GPS_RTK = GPS_Sim(PosVel, Rate, R_b2i, t);
